simulink model "ENEL441LabModel"  (R2012b)
settings: Solver=ode45  StartTime=0.0  StopTime=10.0  RelTol=1e-3
libraries: simulink x1
settings Model: Creator=kyle  LastModifiedBy=kyle

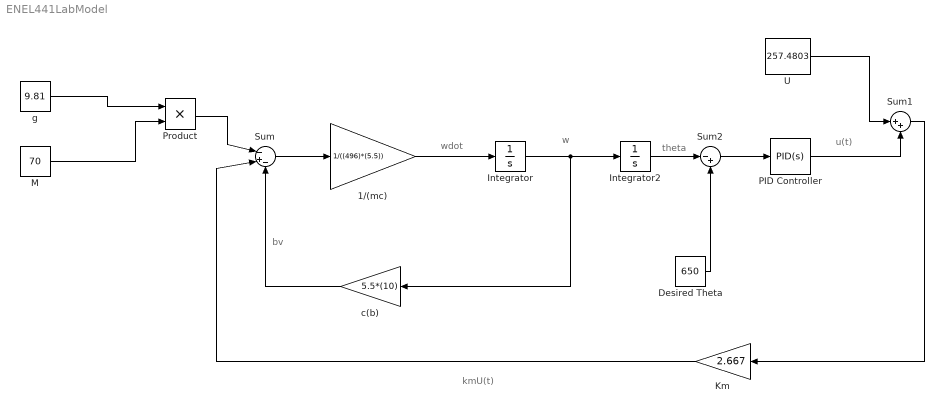
== system ENEL441LabModel ==
  note: u(t)
  note: theta
  note: w
  note: wdot
  note: bv
  note: kmU(t)
  1/(mc) : Gain  Gain=1/((496)*(5.5))
  Desired Theta : Constant  Value=650
  Integrator : Integrator
  Integrator2 : Integrator
  Km : Gain  Gain=2.667
  M : Constant  Value=70
  PID Controller : simulink/Continuous/PID Controller  Controller=PID  TimeDomain=Continuous-time  SampleTime=1  IntegratorMethod=Forward Euler  FilterMethod=Forward Euler  Form=Parallel  P=(496*5.5)/(2.667)  I=10*5.5/2.667  D=0  N=100  InitialConditionSource=internal  InitialConditionForIntegrator=0  InitialConditionForFilter=0  ExternalReset=none  LimitOutput=off  UpperSaturationLimit=inf  LowerSaturationLimit=-inf  LinearizeAsGain=on  AntiWindupMode=none  Kb=1  TrackingMode=off  Kt=1  PParamMin=[]  PParamMax=[]  IParamMin=[]  IParamMax=[]  DParamMin=[]  DParamMax=[]  NParamMin=[]  NParamMax=[]  KbParamMin=[]  KbParamMax=[]  KtParamMin=[]  KtParamMax=[]  POutMin=[]  POutMax=[]  IOutMin=[]  IOutMax=[]  DOutMin=[]  DOutMax=[]  NOutMin=[]  NOutMax=[]  KbOutMin=[]  KbOutMax=[]  KtOutMin=[]  KtOutMax=[]  IntegratorOutMin=[]  IntegratorOutMax=[]  FilterOutMin=[]  FilterOutMax=[]  SumOutMin=[]  SumOutMax=[]  SumI1OutMin=[]  SumI1OutMax=[]  SumI2OutMin=[]  SumI2OutMax=[]  SumI3OutMin=[]  SumI3OutMax=[]  SumDOutMin=[]  SumDOutMax=[]  SaturationOutMin=[]  SaturationOutMax=[]  IntegratorContinuousStateAttributes=''  IntegratorStateMustResolveToSignalObject=off  IntegratorRTWStateStorageClass=Auto  FilterContinuousStateAttributes=''  FilterStateMustResolveToSignalObject=off  FilterRTWStateStorageClass=Auto
  Product : Product  RndMeth=Zero
  Sum : Sum  Inputs=|-+-
  Sum1 : Sum  Inputs=|++
  Sum2 : Sum  Inputs=|-+
  U : Constant  Value=257.4803
  c(b) : Gain  Gain=5.5*(10)
  g : Constant  Value=9.81
  wires:
  Product/1 -> Sum/1
  Sum1/1 -> Km/1
  Km/1 -> Sum/2
  g/1 -> Product/1
  M/1 -> Product/2
  c(b)/1 -> Sum/3
  U/1 -> Sum1/1
  Sum/1 -> 1/(mc)/1
  1/(mc)/1 -> Integrator/1
  Integrator/1 -> Integrator2/1, c(b)/1
  PID Controller/1 -> Sum1/2
  Integrator2/1 -> Sum2/1
  Desired Theta/1 -> Sum2/2
  Sum2/1 -> PID Controller/1
